simulink model "MPPT_solar_sim"  (R2019b)
settings: Solver=VariableStepAuto  StartTime=0.0  StopTime=5.5  RelTol=1e-3
undefined symbols (not defined in the file or in its folder): sigbuilder_block
libraries: powerlib x27, powerlib_meascontrol x2, re_lib x1
settings Model: Creator=root  LastModifiedBy=Gabriel

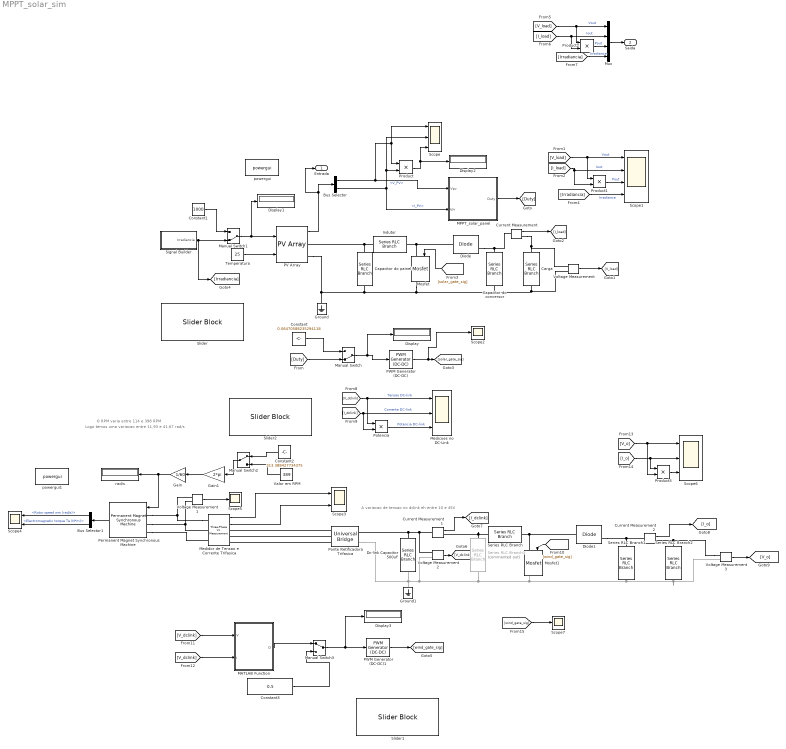
== system MPPT_solar_sim ==
  note: O RPM varia entre 114 e 398 RPM
  note: A variacao de tensao no dclink eh entre 10 e 45V
  note: Logo temos uma variacao entre 11,93 e 41,67 rad/s
  Bus Selector : BusSelector  OutputSignals=V_PV,I_PV
  Bus Selector1 : BusSelector  OutputSignals=Rotor speed wm (rad/s),Electromagnetic torque Te (N*m)
  Capacitor do conversor : powerlib/Elements/Series RLC Branch  LConnTagsString=__new0  RConnTagsString=__new0  BranchType=C  Resistance=1e-4  Inductance=1e-3  SetiL0=off  InitialCurrent=0  Capacitance=1000e-6  Setx0=off  InitialVoltage=0  Measurements=None
      settings: SourceProductName=Simscape Electrical
  Capacitor do painel : powerlib/Elements/Series RLC Branch  LConnTagsString=__new0  RConnTagsString=__new0  BranchType=C  Resistance=1e-4  Inductance=1e-3  SetiL0=off  InitialCurrent=0  Capacitance=100e-6  Setx0=off  InitialVoltage=0  Measurements=None
      settings: SourceProductName=Simscape Electrical
  "Carga " : powerlib/Elements/Series RLC Branch  LConnTagsString=__new0  RConnTagsString=__new0  BranchType=R  Resistance=10  Inductance=1e-3  SetiL0=off  InitialCurrent=0  Capacitance=20e-6  Setx0=off  InitialVoltage=0  Measurements=None
      settings: SourceProductName=Simscape Electrical
  Constant : Constant  Value=0.06470588235294118
  Constant1 : Constant  Value=1000
  Constant2 : Constant  Value=313.388427734375
  Constant3 : Constant  Value=0.5
  Current Measurement : powerlib/Measurements/Current Measurement  PhasorSimulation=off  OutputType=Complex  PSBequivalent=0
      settings: SourceProductName=Simscape Electrical
  Current Measurement1 : powerlib/Measurements/Current Measurement  PhasorSimulation=off  OutputType=Complex  PSBequivalent=0
      settings: SourceProductName=Simscape Electrical
  Current Measurement2 : powerlib/Measurements/Current Measurement  PhasorSimulation=off  OutputType=Complex  PSBequivalent=0
      settings: SourceProductName=Simscape Electrical
  Dc-link Capacitor 500uF : powerlib/Elements/Series RLC Branch  LConnTagsString=__new0  RConnTagsString=__new0  BranchType=C  Resistance=1  Inductance=1e-3  SetiL0=off  InitialCurrent=0  Capacitance=1000e-6  Setx0=off  InitialVoltage=0  Measurements=None
      settings: SourceProductName=Simscape Electrical
  Diode : powerlib/Power Electronics/Diode  Ron=0.001  Lon=0  Vf=0.8  IC=0  UseSnubber=0  Rs=500  Cs=250e-9  Measurements=on
      settings: SourceProductName=Simscape Electrical
  Diode1 : powerlib/Power Electronics/Diode  Ron=0.001  Lon=0  Vf=0.7  IC=0  UseSnubber=0  Rs=500  Cs=250e-9  Measurements=on
      settings: SourceProductName=Simscape Electrical
  Display{,1..3} (4 alike) : Display
  Gain : Gain  Gain=1/60
  Gain1 : Gain  Gain=2*pi
  Ground : powerlib/Elements/Ground  LConnTagsString=a
      settings: SourceProductName=Simscape Electrical
  Ground1 : powerlib/Elements/Ground  LConnTagsString=a
      settings: SourceProductName=Simscape Electrical
  Indutor : powerlib/Elements/Series RLC Branch  LConnTagsString=__new0  RConnTagsString=__new0  BranchType=L  Resistance=1e-4  Inductance=235e-6  SetiL0=off  InitialCurrent=0  Capacitance=100e-6  Setx0=off  InitialVoltage=0  Measurements=None
      settings: SourceProductName=Simscape Electrical
  MATLAB Function : MATLAB Function  TreatAsAtomicUnit=on
  "MPPT_solar_panel " : MATLAB Function  TreatAsAtomicUnit=on
  Manual Switch : ManualSwitch  CurrentSetting=0
  Manual Switch1 : ManualSwitch  CurrentSetting=0
  Manual Switch2 : ManualSwitch
  Manual Switch3 : ManualSwitch
  Medicoes no DC-Link : Scope  NumInputPorts=3
  Medidor de Tensao e Corrente Trifasica : powerlib/Measurements/Three-Phase V-I Measurement  VoltageMeasurement=phase-to-ground  SetLabelV=off  LabelV=Vabc  Vpu=off  VpuLL=off  CurrentMeasurement=yes  SetLabelI=off  LabelI=Iabc  Ipu=off  Pbase=100e6  Vbase=500e3  OutputType=Complex  PhasorSimulation=off  PSBequivalent=0
      settings: SourceProductName=Simscape Electrical
  Mosfet : powerlib/Power Electronics/Mosfet  Ron=0.1  Lon=0  Rd=0.01  Vfd=0  IC=0  Rs=1e5  Cs=inf  Measurements=on
      settings: SourceProductName=Simscape Electrical
  Mosfet1 : powerlib/Power Electronics/Mosfet  Ron=0.1  Lon=0  Rd=0.01  Vfd=0  IC=0  Rs=1e5  Cs=inf  Measurements=on
      settings: SourceProductName=Simscape Electrical
  Mux : Mux
  PV Array : re_lib/Solar/PV Array  Npar=1  Nser=1  PlotType=one module @ 25 deg.C & specified irradiances  S_vec="[ 1000  800  600 400 200]"  Temp_C_vec="[ 45 25  ]"  ModuleName=User-defined  PlotWhenSelected=off  Pm=400.488  Ncell=60  Voc=48.70  Isc=10.79  Vm=40.70  Im=9.84  beta_Voc_pc=-0.289  alpha_Isc_pc=0.051  beta_Voc=-0.14074  alpha_Isc=0.0055029  IL=10.8217  I0=2.2788e-11  nI=1.1776  Rsh=79.7466  Rs=0.23394  BAL=on  Tc=1e-6  Tfilter=1e-3
      settings: SourceProductName=Simscape Electrical
  PWM Generator (DC-DC) : powerlib_meascontrol/Pulse & Signal Generators/PWM Generator (DC-DC)  Fsw=30e3  Ts=0
      settings: SourceProductName=Simscape Electrical
  PWM Generator (DC-DC)1 : powerlib_meascontrol/Pulse & Signal Generators/PWM Generator (DC-DC)  Fsw=50e3  Ts=0
      settings: SourceProductName=Simscape Electrical
  "Permanent Magnet Synchronous Machine " : powerlib/Machines/Permanent Magnet Synchronous Machine  NbPhases=3  FluxDistribution=Sinusoidal  RotorType=Round  MechanicalLoad=Speed w  PresetModel=No  ShowDetailedParameters=on  MeasurementBus=off  Resistance=0.18  Inductance=8.5e-3  dqInductances=[8.5e-3,8.5e-3]  La=0.000835  MachineConstant=Flux linkage established by magnets (V.s)  Flux=0.186667  VoltageCst=101.5729  TorqueCst=0.84  Flat=120  Mechanical=[0.00038 0.000303448 8]  PolePairs=3  InitialConditions=[0,0, 0,0]  InitialConditions5ph=[0 0 0 0 0 0]  RefAngle=90 degrees behind phase A axis (modified Park)  IterativeDiscreteModel=Trapezoidal non iterative  TsBlock=-1  TsPowergui=0
  Ponte Retificadora Trifasica : powerlib/Power Electronics/Universal Bridge  Arms=3  SnubberResistance=1e4  SnubberCapacitance=100e-6  Device=Diodes  Ron=1e-5  Lon=0  ForwardVoltages="[  0  0  ]"  ForwardVoltage=0  GTOparameters=[ 10e-6 , 20e-6 ]  IGBTparameters=[ 1e-6 , 2e-6 ]  Measurements=None  Measurements_2=None  converterType=Rectifier
      settings: SourceProductName=Simscape Electrical
  Potencia : Product
  Product{,1..3} (4 alike) : Product
  Scope : Scope  NumInputPorts=3
  Scope1 : Scope  NumInputPorts=4
  Scope2 : Scope
  Scope3 : Scope  NumInputPorts=2
  Scope4 : Scope  NumInputPorts=2
  Scope5 : Scope
  Scope6 : Scope  NumInputPorts=3
  Scope7 : Scope
  Series RLC Branch : powerlib/Elements/Series RLC Branch  LConnTagsString=__new0  RConnTagsString=__new0  BranchType=L  Resistance=1  Inductance=2.7e-3  SetiL0=off  InitialCurrent=0  Capacitance=1e-6  Setx0=off  InitialVoltage=0  Measurements=None
      settings: SourceProductName=Simscape Electrical
  Series RLC Branch1 : powerlib/Elements/Series RLC Branch  LConnTagsString=__new0  RConnTagsString=__new0  BranchType=RC  Resistance=1e-4  Inductance=1e-3  SetiL0=off  InitialCurrent=0  Capacitance=1000e-6  Setx0=off  InitialVoltage=0  Measurements=None
      settings: SourceProductName=Simscape Electrical
  Series RLC Branch2 : powerlib/Elements/Series RLC Branch  LConnTagsString=__new0  RConnTagsString=__new0  BranchType=R  Resistance=10  Inductance=1e-3  SetiL0=off  InitialCurrent=0  Capacitance=1000e-6  Setx0=off  InitialVoltage=0  Measurements=None
      settings: SourceProductName=Simscape Electrical
  Series RLC Branch3 : powerlib/Elements/Series RLC Branch  Commented=on  LConnTagsString=__new0  RConnTagsString=__new0  BranchType=R  Resistance=10  Inductance=1e-3  SetiL0=off  InitialCurrent=0  Capacitance=1000e-6  Setx0=off  InitialVoltage=0  Measurements=None
      settings: SourceProductName=Simscape Electrical
  Signal Builder : Subsystem  Tag=STV Subsys  LoadFcn=sigbuilder_block('load');  StartFcn=sigbuilder_block('start');  StopFcn=sigbuilder_block('stop');  ClipboardFcn=sigbuilder_block('clipboard');  mask(Sigbuilder block){tuvar=[0:10]}
      mask help: Simulink:masks:SigbuilderBlock_MD
      mask init:
      | if ~strcmp(get_param(bdroot(gcbh),'SimulationStatus'),'stopped') tuvar = sigbuilder_block('maskInit'); end
      settings: CopyFcn=sigbuilder_block('copy');  DeleteFcn=sigbuilder_block('delete');  ModelCloseFcn=sigbuilder_block('modelClose');  PreSaveFcn=sigbuilder_block('preSave');  PauseFcn=sigbuilder_block('pause');  ContinueFcn=sigbuilder_block('continue');  NameChangeFcn=sigbuilder_block('namechange');  OpenFcn=sigbuilder_block('open',[0 0 1868.11 814.378 ]);  CloseFcn=sigbuilder_block('close');
      mask Display: plot(0, 0, 100, 100,[2, 2, 32, 32, 2], [68, 8, 8, 68, 68],[32, 2], [38, 38], [32, 19, 2],[53, 60, 44], [32, 17, 17, 2],[16, 16, 31, 31]);txt = getActiveGroup(gcbh);text(2, 100, txt,'verticalAlignment', 'top');
  Slider : SliderBlock  ScaleMax=1
  Slider1 : SliderBlock  ScaleMax=1
  Slider2 : SliderBlock  ScaleMin=114  ScaleMax=389
  "Temperatura " : Constant  Value=25
  Valor em RPM : Constant  Value=389
  Voltage Measurement{,1..3} (4 alike) : powerlib/Measurements/Voltage Measurement  PhasorSimulation=off  OutputType=Complex  PSBequivalent=0
      settings: SourceProductName=Simscape Electrical
  powergui : powerlib/powergui  Priority=1  SimulationMode=Discrete  SampleTime=1e-6  frequency=60  Iterations=50  frequencyindice=0  Pbase=100e6  ErrMax=1e-4  UnitsV=kV  UnitsW=MW  buscounter=0  FunctionMessages=off  echomessages=off  EnableUseOfTLC=off  CurrentSourceSwitches=off  DisableSnubberDevices=off  DisableRonSwitches=off  DisableVfSwitches=off  DisplayEquations=off  AutomaticDiscreteSolvers=off  SolverType=Tustin/Backward Euler (TBE)  Interpol=off  ExternalGateDelay=off  methode=off  Ts=100  x0status=blocks  SPID=on  SwTol=0  HookPort=off  NonlinearTolerance=1e-4  nMaxIteration=100  ContinueOnMaxIteration=off  RestoreLinks=warning  ResistiveCurrentMeasurement=off  Frange=[0:2:500]  Ylog=off  Xlog=on  ShowGrid=off  save=off  variable=ZData  structure=0  ZoomFFT=off  StartTime=0.0  cycles=1  DisplayStyle=1  fundamental=60  FreqAxis=off  MaxFrequency=1000  frequencyindicesteady=1  RmsSteady=1  display=off
      settings: SourceProductName=Simscape Electrical
  powergui1 : powerlib/powergui  Priority=1  SimulationMode=Discrete  SampleTime=10e-6  frequency=60  Iterations=50  frequencyindice=0  Pbase=100e6  ErrMax=1e-4  UnitsV=kV  UnitsW=MW  buscounter=0  FunctionMessages=off  echomessages=off  EnableUseOfTLC=off  CurrentSourceSwitches=off  DisableSnubberDevices=off  DisableRonSwitches=off  DisableVfSwitches=off  DisplayEquations=off  AutomaticDiscreteSolvers=off  SolverType=Tustin/Backward Euler (TBE)  Interpol=off  ExternalGateDelay=off  methode=off  Ts=100  x0status=blocks  SPID=on  SwTol=0  HookPort=off  NonlinearTolerance=1e-4  nMaxIteration=100  ContinueOnMaxIteration=off  RestoreLinks=warning  ResistiveCurrentMeasurement=off  Frange=[0:2:500]  Ylog=off  Xlog=on  ShowGrid=off  save=off  variable=ZData  structure=0  ZoomFFT=off  StartTime=0.0  cycles=1  DisplayStyle=1  fundamental=60  FreqAxis=off  MaxFrequency=1000  frequencyindicesteady=1  RmsSteady=1  display=off
      settings: SourceProductName=Simscape Electrical
  rad/s : Display
  " Entrada" : Outport
  Saida : Outport  Port=2
  wires:
  Bus Selector/1 -> "MPPT_solar_panel "/1(Vpv), Product/1, Scope/1  "<V_PV>"
  Bus Selector/2 -> "MPPT_solar_panel "/2(Ipv), Scope/2, Product/2  "<I_PV>"
  PV Array/1 -> Bus Selector/1, " Entrada"/1
  Voltage Measurement/1 -> [V_load]
  Current Measurement/1 -> [I_load]
  [V_load] -> Product1/1, Scope1/1  "Vout"
  [I_load] -> Scope1/2, Product1/2  "Iout"
  PWM Generator (DC-DC)/1 -> Scope2/1, [solar_gate_sig]
  Product/1 -> Display2/1, Scope/3
  [Duty] -> Manual Switch/2
  Manual Switch/1 -> Display/1, PWM Generator (DC-DC)/1
  Constant/1 -> Manual Switch/1
  Product1/1 -> Scope1/3  "Pout"
  Manual Switch1/1 -> Display1/1, PV Array/1
  Constant1/1 -> Manual Switch1/1
  [solar_gate_sig] -> Mosfet/1
  "MPPT_solar_panel "/1(Duty) -> [Duty]
  Signal Builder/1(Irradiancia) -> [Irradiancia], Manual Switch1/2
  "Temperatura "/1 -> PV Array/2
  [Irradiancia] -> Scope1/4  "Irradiance"
  Mux/1 -> Saida/1
  [V_load] -> Product2/1, Mux/1  "Vout"
  [I_load] -> Product2/2, Mux/2  "Iout"
  Product2/1 -> Mux/3  "Pout"
  [Irradiancia] -> Mux/4  "Irradiance"
  Valor em RPM/1 -> Manual Switch2/2
  Constant2/1 -> Manual Switch2/1
  [V_dclink] -> MATLAB Function/2(I)
  Medidor de Tensao e Corrente Trifasica/1 -> Scope3/1
  Manual Switch2/1 -> Gain1/1
  [I_o] -> Product3/1, Scope6/2
  [wind_gate_sig] -> Scope7/1
  MATLAB Function/1(D) -> Manual Switch3/1
  Constant3/1 -> Manual Switch3/2
  [I_dclink] -> Medicoes no DC-Link/2, Potencia/2  "Corrente DC-link"
  Current Measurement1/1 -> [I_dclink]
  Current Measurement2/1 -> [I_o]
  [V_dclink] -> MATLAB Function/1(V)
  [V_dclink] -> Medicoes no DC-Link/1, Potencia/1  "Tensao DC-link"
  Voltage Measurement3/1 -> [V_o]
  Voltage Measurement2/1 -> [V_dclink]
  [wind_gate_sig] -> Mosfet1/1
  Potencia/1 -> Medicoes no DC-Link/3  "Potencia DC-link"
  [V_o] -> Product3/2, Scope6/1
  Gain1/1 -> Gain/1
  Product3/1 -> Scope6/3
  Gain/1 -> rad/s/1, "Permanent Magnet Synchronous Machine "/1
  Bus Selector1/1 -> Scope4/1  "<Rotor speed wm (rad/s)>"
  PWM Generator (DC-DC)1/1 -> [wind_gate_sig]
  Medidor de Tensao e Corrente Trifasica/2 -> Scope3/2
  Manual Switch3/1 -> Display3/1, PWM Generator (DC-DC)1/1
  Voltage Measurement1/1 -> Scope5/1
  "Permanent Magnet Synchronous Machine "/1 -> Bus Selector1/1
  Bus Selector1/2 -> Scope4/2  "<Electromagnetic torque Te (N*m)>"
  connections:
  PV Array/RConn2 -- Mosfet/RConn1 -- Voltage Measurement/LConn2 -- "Carga "/RConn1 -- Capacitor do conversor/RConn1 -- Capacitor do painel/RConn1 -- Ground/LConn1
  "Carga "/LConn1 -- Voltage Measurement/LConn1 -- Current Measurement/RConn1
  Current Measurement/LConn1 -- Diode/RConn1 -- Capacitor do conversor/LConn1
  Capacitor do painel/LConn1 -- PV Array/RConn1 -- Indutor/RConn1
  Mosfet/LConn1 -- Diode/LConn1 -- Indutor/LConn1
  Current Measurement1/RConn1 -- Series RLC Branch3/LConn1 -- Series RLC Branch/LConn1
  Voltage Measurement2/LConn1 -- Dc-link Capacitor 500uF/LConn1 -- Ponte Retificadora Trifasica/RConn1 -- Current Measurement1/LConn1
  Series RLC Branch3/RConn1 -- Voltage Measurement3/LConn2 -- Series RLC Branch2/RConn1 -- Series RLC Branch1/RConn1 -- Mosfet1/RConn1 -- Ground1/LConn1 -- Ponte Retificadora Trifasica/RConn2 -- Dc-link Capacitor 500uF/RConn1 -- Voltage Measurement2/LConn2
  Voltage Measurement3/LConn1 -- Current Measurement2/RConn1 -- Series RLC Branch2/LConn1
  Series RLC Branch/RConn1 -- Mosfet1/LConn1 -- Diode1/LConn1
  Series RLC Branch1/LConn1 -- Diode1/RConn1 -- Current Measurement2/LConn1
  Voltage Measurement1/LConn2 -- "Permanent Magnet Synchronous Machine "/LConn2 -- Medidor de Tensao e Corrente Trifasica/LConn2
  Medidor de Tensao e Corrente Trifasica/LConn1 -- "Permanent Magnet Synchronous Machine "/LConn1 -- Voltage Measurement1/LConn1
  "Permanent Magnet Synchronous Machine "/LConn3 -- Medidor de Tensao e Corrente Trifasica/LConn3
  Ponte Retificadora Trifasica/LConn1 -- Medidor de Tensao e Corrente Trifasica/RConn1
  Ponte Retificadora Trifasica/LConn2 -- Medidor de Tensao e Corrente Trifasica/RConn2
  Ponte Retificadora Trifasica/LConn3 -- Medidor de Tensao e Corrente Trifasica/RConn3

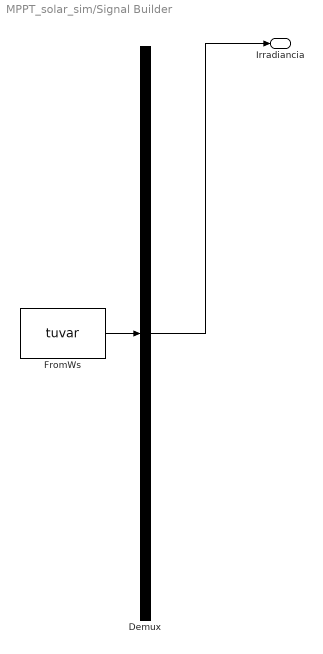
== system MPPT_solar_sim/Signal Builder ==
  Demux : Demux  Tag=STV Demux  Outputs=1
  FromWs : FromWorkspace  Tag=STV FromWs  VariableName=tuvar  SampleTime=0
      SigBuilderData=|
      | common.afterFinalStr = 'Extrapolate'
      | common.sampleTime = 0
      | dataSet.timeRange = [0 10]
      | dataSet.name = 'Group 1'
      | sbobj.Groups.Name = 'Group 1'
      | sbobj.Groups.Signals.Name = 'Irradiancia'
      | sbobj.Groups.Signals.XData = [0 0.5 0.5 1 1 1.5 1.5 2 2 2.5 2.5 3 3 3.5 3.5 4 4 4.5 4.5 5 5 10]
      | sbobj.Groups.Signals.YData = [0 0 200 200 400 400 600 600 800 800 1002 1000 800 800 600 600 400 400 200 200 0 0]
  Irradiancia : Outport  Tag=STV Outport
  wires:
  Demux/1 -> Irradiancia/1
  FromWs/1 -> Demux/1

== matlab function MPPT_solar_sim/MPPT_solar_panel  ==
  data: Vpv input; Duty output; Ipv input
% Codigo para algoritmo MPPT pertubation and observation
% para o painel fotovoltaico.

function Duty = MPPT_solar_panel(Vpv, Ipv)


    %% Declaramos as variaveis do tipo persistent de forma que os valores 
    % fiquem armazenados mesmo com o término da função
    
    persistent Vpv_old Ppv_old Duty_old
    
    % Inicializacao das variaveis
    if isempty(Duty_old)
       Duty_old = 0.5;
       Ppv_old = 0;
       Vpv_old = 0;
    end
    
    Duty_var = 125e-6;           % Delta de variacao a cada iteracao
    
    
    % Calculo do valor de potencia
    
    Ppv = Vpv * Ipv;
    
    %% Inicializacao da comparacao
    
    if ((Ppv - Ppv_old) ~= 0)
       if ((Ppv - Ppv_old) < 0) 
            if ((Vpv - Vpv_old) < 0)
                Duty = Duty_old - Duty_var;
            else 
                Duty = Duty_old + Duty_var;
            end
       else 
           if ((Vpv - Vpv_old) < 0)
                Duty = Duty_old + Duty_var;
           else 
               Duty = Duty_old - Duty_var;
           end
       end
    else 
        
        Duty = Duty_old;
        
    end
    
    if (Duty > 1)
        Duty = 1.0;
    elseif Duty < 0
        Duty = 0.0;
    end 
    
    Ppv_old = Ppv;
    Vpv_old = Vpv;
    Duty_old = Duty;    
end

== matlab function MPPT_solar_sim/MATLAB Function ==
  data: V input; D output; I input
% PO algoritm for wind power system

% This function receive voltage and current from dc link
% Dc link is the point following the filter capacitor for rectifier


function D = MPPT_WDS(V, I)


% primeiro declaramos as variaveis

persistent V_old P_old;

if isempty(P_old)
    V_old= 50;
    P_old=100;
end

P = V*I;

dP = P-P_old;
dv = V-V_old;

delta = 0.01;

if (dP~=0)
    if (dP>0)
        if (dv>0)
            V_mppt = V_old + delta;
        else 
            V_mppt = V_old - delta;
        end
    else
        if (dv>0)
            V_mppt = V_old - delta;
        else
            V_mppt = V_old + delta;
        end
    end
else 
    V_mppt = V_old;
end

D = 1- V_mppt/100;

P_old = P;
V_old = V_mppt;
end
